simulink subsystem "controller"  (R2024b)
settings: Solver=VariableStepAuto  StartTime=0.0  StopTime=10.0  RelTol=1e-3
values from neighbouring files (symbols this model uses):
  C_out = 12    [dados_conversor.m]
  L = 80e-3    (= 0.08)    [KF_obs_test.m]    (also in RLSF_test.m = L_nom*ones(n_phases, 1); backup_2407_2.m = L_nom*ones(n_phases, 1); controller_mtlbfun.m = L_nom*ones(n_phases, 1); dados_conversor.m = 80)
  R_L = 100    [dados_conversor.m]
  Ts = 0.001    [boost_data.mat]
  Vout_ref = 96    [MRAC2_test.m]    (also in MRAC_test.m; RLSF_test.m)
undefined symbols (not defined in the file or in its folder): Kj, Kr
settings Model: Creator=eric  LastModifiedBy=eric

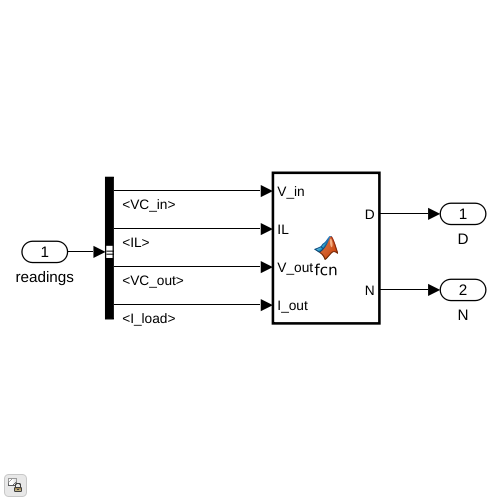
[thumbnail: Simulink's stored preview of the top-level diagram]
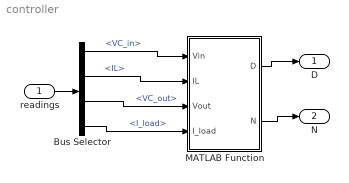
== system controller ==
  readings : Inport
  Bus Selector : BusSelector  OutputSignals=VC_in,IL,VC_out,I_load
  MATLAB Function : MATLAB Function  TreatAsAtomicUnit=on  SystemSampleTime=Ts
  D : Outport
  N : Outport  Port=2
  wires:
  MATLAB Function/2(N) -> N/1
  MATLAB Function/1(D) -> D/1
  readings/1 -> Bus Selector/1
  Bus Selector/1 -> MATLAB Function/1(Vin)  "<VC_in>"
  Bus Selector/2 -> MATLAB Function/2(IL)  "<IL>"
  Bus Selector/3 -> MATLAB Function/3(Vout)  "<VC_out>"
  Bus Selector/4 -> MATLAB Function/4(I_load)  "<I_load>"

== matlab function controller/MATLAB Function ==
  data: D output; N output; Vin input; IL input; Vout input; I_load input; C_out parameter; L parameter; R_L parameter; Kj parameter; Kr parameter; Vout_ref parameter
function [D, N] = fcn(Vin, IL, Vout, I_load, C_out, L, R_L, Kj, Kr, Vout_ref)
    N = 35;

    IL1 = IL(1); IL2 = IL(2); IL3 = IL(3);
    IL_ref = Vout*I_load/sum(IL); % Conservaçao de energia/potencia

    IL_ref_dot = 0;

    if Vout > Vin

        d_num = function_d_num(C_out, IL1, IL2, IL3, IL_ref, IL_ref_dot, I_load, Kj, Kr, L, R_L, Vin, Vout, Vout_ref);
        d_den = function_d_den(C_out, IL1, IL2, IL3, L, Vout);
    
        D = d_num./d_den;
        D = max(0, min(D, 1));
    else
        D = zeros(3, 1);
    end
end
